simulink model "V2G_Gajduk"  (R2017a)
settings: Solver=ode23t  StartTime=0.0  StopTime=10  RelTol=1e-3
values from neighbouring files (symbols this model uses):
  C_Vdc = 100*18e-3    (= 1.8)    [main_v2gg2v.m]
  Cf = 10*165e-6    (= 0.00165)    [main_v2gg2v.m]
  D = 20    [main_v2gg2v.m]
  E1 = 1.07364213042869    (= 1.07364213043)    [main_v2gg2v.m]
  E2 = 1.05726676017896    (= 1.05726676018)    [main_v2gg2v.m]
  E3 = 1.05298913370226    (= 1.0529891337)    [main_v2gg2v.m]
  f_grid = 50    [main_v2gg2v.m]
  H1 = 10    [main_v2gg2v.m]
  H2 = 15    [main_v2gg2v.m]
  H3 = 60    [main_v2gg2v.m]
  h_PEV = -2000    [main_v2gg2v.m]
  Ibat_ref = -200    [main_v2gg2v.m]
  Ibatfault_ref = 200    [main_v2gg2v.m]
  Ki_CC = 1    [main_v2gg2v.m]
  Ki_inner = 5000    [main_v2gg2v.m]
  Ki_outer = 10000    [main_v2gg2v.m]
  Ki_PLL = 10000    [main_v2gg2v.m]
  Kp_CC = 10    [main_v2gg2v.m]
  Kp_inner = 100    [main_v2gg2v.m]
  Kp_outer = 250    [main_v2gg2v.m]
  Kp_PLL = 100    [main_v2gg2v.m]
  Lbat = 2e-3    (= 0.002)    [main_v2gg2v.m]
  Lgrid = 1/10*0.69e-3    (= 6.9e-05)    [main_v2gg2v.m]
  Linv = 1/10*0.48e-3    (= 4.8e-05)    [main_v2gg2v.m]
  LowSat_CC = 0    [main_v2gg2v.m]
  omega = 2*pi*f_grid    (= 314.159265359)    [main_v2gg2v.m]
  Pm1 = 2.49    [main_v2gg2v.m]
  Pm2 = 4.21    [main_v2gg2v.m]
  Pm3 = 8.20    (= 8.2)    [main_v2gg2v.m]
  Rd = 1.31    [main_v2gg2v.m]
  S1pu = (1.5 + .45j)    [main_v2gg2v.m]
  S2pu = (1.0 + .3j)    [main_v2gg2v.m]
  S3pu = (12.4 + 2.5j)    [main_v2gg2v.m]
  Sbase = 1e6    (= 1000000)    [main_v2gg2v.m]
  Snom_trafo = 1050e6    (= 1050000000)    [main_v2gg2v.m]
  t_fault_end = t_fault_start + FCT    (= 0.723)    [main_v2gg2v.m]
  t_fault_start = 0.5    [main_v2gg2v.m]
  Ts = 1e-5    (= 1e-05)    [main_v2gg2v.m]
  UpSat_CC = 1    [main_v2gg2v.m]
  Vbase = 345e3    (= 345000)    [main_v2gg2v.m]
  Vdc_ref = 1.5e3    (= 1500)    [main_v2gg2v.m]
  Vfault_thresh = 455    [main_v2gg2v.m]
undefined symbols (not defined in the file or in its folder): D1, Delta, Ion, L12, L13, L23, Lbuckboost, Lithium, R_Vdc, Rbuckboost
libraries: powerlib x175, powerlib_meascontrol x55, simulink x45, electricdrivelib x30, dspstat3 x3
(part 5 of 5)

== system V2G_Gajduk/V2G-G2V-3/5 Charging Stations/Charging Station4 ==
  Ibat_ref : Inport
  Battery : electricdrivelib/Extra Sources/Battery  BatType=Lithium-Ion  ShowTempParam=off  ThermalPreset=no  ShowAgeParam=off  NomV=Batt_Vnom  NomQ=Batt_Ah  SOC=Batt_InitSOC  Batt_Tr=Batt_RespTime  PresetModel=on  MaxQ=35  MinV=300  FullV=465.5949  Dis_rate=15.2174  R=0.11429  Normal_OP=31.6522  expZone="[432.1543      1.719565]"  current=[6.5 13 32.5]  Units=Time  Tci=20  NomT=20  T2=-30  MaxQ2=4.8  FullV2=7.1  Normal_OP2=5.655  expZone2="[6.58           1]"  Rca=0.6  ti=2000  Dp=0  Neq0=0  Tsim=1e6  Ta1=25  Qeol=5.4*0.9  Reol=0.013333*1.2  Char_age=[2.3478, 3]  Dis_age=[2.3478, 10]  N1=1500  N2=10500  N3=1000  N4=1400  Ta2=45  N5=950
  Bus Selector : BusSelector  OutputSignals=SOC (%),Current (A),Voltage (V)
  Logical Operator : Logic  Operator=NOT  AllPortsSameDT=off  OutDataTypeStr=boolean
  Mosfet : powerlib/Power Electronics/Mosfet  Ron=0.1  Lon=0  Rd=0.01  Vfd=0  IC=0  Rs=1e5  Cs=inf  Measurements=off
  Mosfet1 : powerlib/Power Electronics/Mosfet  Ron=0.1  Lon=0  Rd=0.01  Vfd=0  IC=0  Rs=1e5  Cs=inf  Measurements=off
  PID Controller4 : simulink/Continuous/PID Controller  Controller=PI  TimeDomain=Continuous-time  SampleTime=-1  IntegratorMethod=Forward Euler  FilterMethod=Forward Euler  Form=Parallel  UseFilter=on  ControllerParametersSource=internal  P=Kp_CC  I=Ki_CC  D=0  N=100  InitialConditionSource=internal  InitialConditionForIntegrator=0  InitialConditionForFilter=0  ExternalReset=none  ZeroCross=off  LimitOutput=on  UpperSaturationLimit=UpSat_CC  LowerSaturationLimit=LowSat_CC  LinearizeAsGain=on  AntiWindupMode=none  Kb=1  TrackingMode=off  Kt=1  PParamMin=[]  PParamMax=[]  IParamMin=[]  IParamMax=[]  DParamMin=[]  DParamMax=[]  NParamMin=[]  NParamMax=[]  KbParamMin=[]  KbParamMax=[]  KtParamMin=[]  KtParamMax=[]  POutMin=[]  POutMax=[]  IOutMin=[]  IOutMax=[]  DOutMin=[]  DOutMax=[]  NOutMin=[]  NOutMax=[]  KbOutMin=[]  KbOutMax=[]  KtOutMin=[]  KtOutMax=[]  IntegratorOutMin=[]  IntegratorOutMax=[]  FilterOutMin=[]  FilterOutMax=[]  SumOutMin=[]  SumOutMax=[]  SumI1OutMin=[]  SumI1OutMax=[]  SumI2OutMin=[]  SumI2OutMax=[]  SumI3OutMin=[]  SumI3OutMax=[]  SumDOutMin=[]  SumDOutMax=[]  SaturationOutMin=[]  SaturationOutMax=[]  IntegratorContinuousStateAttributes=''  IntegratorStateMustResolveToSignalObject=off  IntegratorRTWStateStorageClass=Auto  FilterContinuousStateAttributes=''  FilterStateMustResolveToSignalObject=off  FilterRTWStateStorageClass=Auto  DifferentiatorICPrevScaledInput=0  DifferentiatorOutMin=[]  DifferentiatorOutMax=[]  InitialConditionSetting=State (most efficient)
  PWM Generator (DC-DC) : powerlib_meascontrol/Pulse & Signal Generators/PWM Generator (DC-DC)  Fsw=f_SW  Ts=0
  Series RLC Branch9 : powerlib/Elements/Series RLC Branch  LConnTagsString=__new0  RConnTagsString=__new0  BranchType=L  Resistance=Rbuckboost  Inductance=Lbat  SetiL0=off  InitialCurrent=0  Capacitance=1e-6  Setx0=off  InitialVoltage=0  Measurements=None
  Sum8 : Sum  Inputs=|+-
  Terminator{,1..3} (4 alike) : Terminator
  VDC+ : PMIOPort  Port=1  Side=Left
  VDC- : PMIOPort  Port=2  Side=Left
  wires:
  Bus Selector/3 -> Terminator3/1  "<Voltage (V)>"
  Bus Selector/2 -> Terminator2/1, [Ibat]  "<Current (A)>"
  [Buck] -> Mosfet/1
  Battery/1 -> Terminator/1, Bus Selector/1
  [Boost] -> Mosfet1/1
  Bus Selector/1 -> Terminator1/1  "<SOC (%)>"
  Logical Operator/1 -> [Boost]
  Ibat_ref/1 -> Sum8/2
  PID Controller4/1 -> PWM Generator (DC-DC)/1
  [Ibat] -> Sum8/1
  Sum8/1 -> PID Controller4/1
  PWM Generator (DC-DC)/1 -> Logical Operator/1, [Buck]
  connections:
  VDC-/RConn1 -- Battery/LConn2 -- Mosfet1/RConn1
  Mosfet/LConn1 -- VDC+/RConn1
  Mosfet1/LConn1 -- Series RLC Branch9/RConn1 -- Mosfet/RConn1
  Battery/LConn1 -- Series RLC Branch9/LConn1

== system V2G_Gajduk/V2G-G2V-3/5 Charging Stations/Charging Station5 ==
  Ibat_ref : Inport
  Battery : electricdrivelib/Extra Sources/Battery  BatType=Lithium-Ion  ShowTempParam=off  ThermalPreset=no  ShowAgeParam=off  NomV=Batt_Vnom  NomQ=Batt_Ah  SOC=Batt_InitSOC  Batt_Tr=Batt_RespTime  PresetModel=on  MaxQ=35  MinV=300  FullV=465.5949  Dis_rate=15.2174  R=0.11429  Normal_OP=31.6522  expZone="[432.1543      1.719565]"  current=[6.5 13 32.5]  Units=Time  Tci=20  NomT=20  T2=-30  MaxQ2=4.8  FullV2=7.1  Normal_OP2=5.655  expZone2="[6.58           1]"  Rca=0.6  ti=2000  Dp=0  Neq0=0  Tsim=1e6  Ta1=25  Qeol=5.4*0.9  Reol=0.013333*1.2  Char_age=[2.3478, 3]  Dis_age=[2.3478, 10]  N1=1500  N2=10500  N3=1000  N4=1400  Ta2=45  N5=950
  Bus Selector : BusSelector  OutputSignals=SOC (%),Current (A),Voltage (V)
  Logical Operator : Logic  Operator=NOT  AllPortsSameDT=off  OutDataTypeStr=boolean
  Mosfet : powerlib/Power Electronics/Mosfet  Ron=0.1  Lon=0  Rd=0.01  Vfd=0  IC=0  Rs=1e5  Cs=inf  Measurements=off
  Mosfet1 : powerlib/Power Electronics/Mosfet  Ron=0.1  Lon=0  Rd=0.01  Vfd=0  IC=0  Rs=1e5  Cs=inf  Measurements=off
  PID Controller4 : simulink/Continuous/PID Controller  Controller=PI  TimeDomain=Continuous-time  SampleTime=-1  IntegratorMethod=Forward Euler  FilterMethod=Forward Euler  Form=Parallel  UseFilter=on  ControllerParametersSource=internal  P=Kp_CC  I=Ki_CC  D=0  N=100  InitialConditionSource=internal  InitialConditionForIntegrator=0  InitialConditionForFilter=0  ExternalReset=none  ZeroCross=off  LimitOutput=on  UpperSaturationLimit=UpSat_CC  LowerSaturationLimit=LowSat_CC  LinearizeAsGain=on  AntiWindupMode=none  Kb=1  TrackingMode=off  Kt=1  PParamMin=[]  PParamMax=[]  IParamMin=[]  IParamMax=[]  DParamMin=[]  DParamMax=[]  NParamMin=[]  NParamMax=[]  KbParamMin=[]  KbParamMax=[]  KtParamMin=[]  KtParamMax=[]  POutMin=[]  POutMax=[]  IOutMin=[]  IOutMax=[]  DOutMin=[]  DOutMax=[]  NOutMin=[]  NOutMax=[]  KbOutMin=[]  KbOutMax=[]  KtOutMin=[]  KtOutMax=[]  IntegratorOutMin=[]  IntegratorOutMax=[]  FilterOutMin=[]  FilterOutMax=[]  SumOutMin=[]  SumOutMax=[]  SumI1OutMin=[]  SumI1OutMax=[]  SumI2OutMin=[]  SumI2OutMax=[]  SumI3OutMin=[]  SumI3OutMax=[]  SumDOutMin=[]  SumDOutMax=[]  SaturationOutMin=[]  SaturationOutMax=[]  IntegratorContinuousStateAttributes=''  IntegratorStateMustResolveToSignalObject=off  IntegratorRTWStateStorageClass=Auto  FilterContinuousStateAttributes=''  FilterStateMustResolveToSignalObject=off  FilterRTWStateStorageClass=Auto  DifferentiatorICPrevScaledInput=0  DifferentiatorOutMin=[]  DifferentiatorOutMax=[]  InitialConditionSetting=State (most efficient)
  PWM Generator (DC-DC) : powerlib_meascontrol/Pulse & Signal Generators/PWM Generator (DC-DC)  Fsw=f_SW  Ts=0
  Series RLC Branch9 : powerlib/Elements/Series RLC Branch  LConnTagsString=__new0  RConnTagsString=__new0  BranchType=L  Resistance=Rbuckboost  Inductance=Lbat  SetiL0=off  InitialCurrent=0  Capacitance=1e-6  Setx0=off  InitialVoltage=0  Measurements=None
  Sum8 : Sum  Inputs=|+-
  Terminator{,1..3} (4 alike) : Terminator
  VDC+ : PMIOPort  Port=1  Side=Left
  VDC- : PMIOPort  Port=2  Side=Left
  wires:
  Bus Selector/3 -> Terminator3/1  "<Voltage (V)>"
  Bus Selector/2 -> Terminator2/1, [Ibat]  "<Current (A)>"
  [Buck] -> Mosfet/1
  Battery/1 -> Terminator/1, Bus Selector/1
  [Boost] -> Mosfet1/1
  Bus Selector/1 -> Terminator1/1  "<SOC (%)>"
  Logical Operator/1 -> [Boost]
  Ibat_ref/1 -> Sum8/2
  PID Controller4/1 -> PWM Generator (DC-DC)/1
  [Ibat] -> Sum8/1
  Sum8/1 -> PID Controller4/1
  PWM Generator (DC-DC)/1 -> Logical Operator/1, [Buck]
  connections:
  VDC-/RConn1 -- Battery/LConn2 -- Mosfet1/RConn1
  Mosfet/LConn1 -- VDC+/RConn1
  Mosfet1/LConn1 -- Series RLC Branch9/RConn1 -- Mosfet/RConn1
  Battery/LConn1 -- Series RLC Branch9/LConn1

== system V2G_Gajduk/V2G-G2V-3/5 Charging Stations/Charging Station6 ==
  Ibat_ref : Inport
  Battery : electricdrivelib/Extra Sources/Battery  BatType=Lithium-Ion  ShowTempParam=off  ThermalPreset=no  ShowAgeParam=off  NomV=Batt_Vnom  NomQ=Batt_Ah  SOC=Batt_InitSOC  Batt_Tr=Batt_RespTime  PresetModel=on  MaxQ=35  MinV=300  FullV=465.5949  Dis_rate=15.2174  R=0.11429  Normal_OP=31.6522  expZone="[432.1543      1.719565]"  current=[6.5 13 32.5]  Units=Time  Tci=20  NomT=20  T2=-30  MaxQ2=4.8  FullV2=7.1  Normal_OP2=5.655  expZone2="[6.58           1]"  Rca=0.6  ti=2000  Dp=0  Neq0=0  Tsim=1e6  Ta1=25  Qeol=5.4*0.9  Reol=0.013333*1.2  Char_age=[2.3478, 3]  Dis_age=[2.3478, 10]  N1=1500  N2=10500  N3=1000  N4=1400  Ta2=45  N5=950
  Bus Selector : BusSelector  OutputSignals=SOC (%),Current (A),Voltage (V)
  Logical Operator : Logic  Operator=NOT  AllPortsSameDT=off  OutDataTypeStr=boolean
  Mosfet : powerlib/Power Electronics/Mosfet  Ron=0.1  Lon=0  Rd=0.01  Vfd=0  IC=0  Rs=1e5  Cs=inf  Measurements=off
  Mosfet1 : powerlib/Power Electronics/Mosfet  Ron=0.1  Lon=0  Rd=0.01  Vfd=0  IC=0  Rs=1e5  Cs=inf  Measurements=off
  PID Controller4 : simulink/Continuous/PID Controller  Controller=PI  TimeDomain=Continuous-time  SampleTime=-1  IntegratorMethod=Forward Euler  FilterMethod=Forward Euler  Form=Parallel  UseFilter=on  ControllerParametersSource=internal  P=Kp_CC  I=Ki_CC  D=0  N=100  InitialConditionSource=internal  InitialConditionForIntegrator=0  InitialConditionForFilter=0  ExternalReset=none  ZeroCross=off  LimitOutput=on  UpperSaturationLimit=UpSat_CC  LowerSaturationLimit=LowSat_CC  LinearizeAsGain=on  AntiWindupMode=none  Kb=1  TrackingMode=off  Kt=1  PParamMin=[]  PParamMax=[]  IParamMin=[]  IParamMax=[]  DParamMin=[]  DParamMax=[]  NParamMin=[]  NParamMax=[]  KbParamMin=[]  KbParamMax=[]  KtParamMin=[]  KtParamMax=[]  POutMin=[]  POutMax=[]  IOutMin=[]  IOutMax=[]  DOutMin=[]  DOutMax=[]  NOutMin=[]  NOutMax=[]  KbOutMin=[]  KbOutMax=[]  KtOutMin=[]  KtOutMax=[]  IntegratorOutMin=[]  IntegratorOutMax=[]  FilterOutMin=[]  FilterOutMax=[]  SumOutMin=[]  SumOutMax=[]  SumI1OutMin=[]  SumI1OutMax=[]  SumI2OutMin=[]  SumI2OutMax=[]  SumI3OutMin=[]  SumI3OutMax=[]  SumDOutMin=[]  SumDOutMax=[]  SaturationOutMin=[]  SaturationOutMax=[]  IntegratorContinuousStateAttributes=''  IntegratorStateMustResolveToSignalObject=off  IntegratorRTWStateStorageClass=Auto  FilterContinuousStateAttributes=''  FilterStateMustResolveToSignalObject=off  FilterRTWStateStorageClass=Auto  DifferentiatorICPrevScaledInput=0  DifferentiatorOutMin=[]  DifferentiatorOutMax=[]  InitialConditionSetting=State (most efficient)
  PWM Generator (DC-DC) : powerlib_meascontrol/Pulse & Signal Generators/PWM Generator (DC-DC)  Fsw=f_SW  Ts=0
  Series RLC Branch9 : powerlib/Elements/Series RLC Branch  LConnTagsString=__new0  RConnTagsString=__new0  BranchType=L  Resistance=Rbuckboost  Inductance=Lbat  SetiL0=off  InitialCurrent=0  Capacitance=1e-6  Setx0=off  InitialVoltage=0  Measurements=None
  Sum8 : Sum  Inputs=|+-
  Terminator{,1..3} (4 alike) : Terminator
  VDC+ : PMIOPort  Port=1  Side=Left
  VDC- : PMIOPort  Port=2  Side=Left
  wires:
  Bus Selector/3 -> Terminator3/1  "<Voltage (V)>"
  Bus Selector/2 -> Terminator2/1, [Ibat]  "<Current (A)>"
  [Buck] -> Mosfet/1
  Battery/1 -> Terminator/1, Bus Selector/1
  [Boost] -> Mosfet1/1
  Bus Selector/1 -> Terminator1/1  "<SOC (%)>"
  Logical Operator/1 -> [Boost]
  Ibat_ref/1 -> Sum8/2
  PID Controller4/1 -> PWM Generator (DC-DC)/1
  [Ibat] -> Sum8/1
  Sum8/1 -> PID Controller4/1
  PWM Generator (DC-DC)/1 -> Logical Operator/1, [Buck]
  connections:
  VDC-/RConn1 -- Battery/LConn2 -- Mosfet1/RConn1
  Mosfet/LConn1 -- VDC+/RConn1
  Mosfet1/LConn1 -- Series RLC Branch9/RConn1 -- Mosfet/RConn1
  Battery/LConn1 -- Series RLC Branch9/LConn1

== system V2G_Gajduk/V2G-G2V-3/5 Charging Stations/Charging Station7 ==
  Ibat_ref : Inport
  Battery : electricdrivelib/Extra Sources/Battery  BatType=Lithium-Ion  ShowTempParam=off  ThermalPreset=no  ShowAgeParam=off  NomV=Batt_Vnom  NomQ=Batt_Ah  SOC=Batt_InitSOC  Batt_Tr=Batt_RespTime  PresetModel=on  MaxQ=35  MinV=300  FullV=465.5949  Dis_rate=15.2174  R=0.11429  Normal_OP=31.6522  expZone="[432.1543      1.719565]"  current=[6.5 13 32.5]  Units=Time  Tci=20  NomT=20  T2=-30  MaxQ2=4.8  FullV2=7.1  Normal_OP2=5.655  expZone2="[6.58           1]"  Rca=0.6  ti=2000  Dp=0  Neq0=0  Tsim=1e6  Ta1=25  Qeol=5.4*0.9  Reol=0.013333*1.2  Char_age=[2.3478, 3]  Dis_age=[2.3478, 10]  N1=1500  N2=10500  N3=1000  N4=1400  Ta2=45  N5=950
  Bus Selector : BusSelector  OutputSignals=SOC (%),Current (A),Voltage (V)
  Logical Operator : Logic  Operator=NOT  AllPortsSameDT=off  OutDataTypeStr=boolean
  Mosfet : powerlib/Power Electronics/Mosfet  Ron=0.1  Lon=0  Rd=0.01  Vfd=0  IC=0  Rs=1e5  Cs=inf  Measurements=off
  Mosfet1 : powerlib/Power Electronics/Mosfet  Ron=0.1  Lon=0  Rd=0.01  Vfd=0  IC=0  Rs=1e5  Cs=inf  Measurements=off
  PID Controller4 : simulink/Continuous/PID Controller  Controller=PI  TimeDomain=Continuous-time  SampleTime=-1  IntegratorMethod=Forward Euler  FilterMethod=Forward Euler  Form=Parallel  UseFilter=on  ControllerParametersSource=internal  P=Kp_CC  I=Ki_CC  D=0  N=100  InitialConditionSource=internal  InitialConditionForIntegrator=0  InitialConditionForFilter=0  ExternalReset=none  ZeroCross=off  LimitOutput=on  UpperSaturationLimit=UpSat_CC  LowerSaturationLimit=LowSat_CC  LinearizeAsGain=on  AntiWindupMode=none  Kb=1  TrackingMode=off  Kt=1  PParamMin=[]  PParamMax=[]  IParamMin=[]  IParamMax=[]  DParamMin=[]  DParamMax=[]  NParamMin=[]  NParamMax=[]  KbParamMin=[]  KbParamMax=[]  KtParamMin=[]  KtParamMax=[]  POutMin=[]  POutMax=[]  IOutMin=[]  IOutMax=[]  DOutMin=[]  DOutMax=[]  NOutMin=[]  NOutMax=[]  KbOutMin=[]  KbOutMax=[]  KtOutMin=[]  KtOutMax=[]  IntegratorOutMin=[]  IntegratorOutMax=[]  FilterOutMin=[]  FilterOutMax=[]  SumOutMin=[]  SumOutMax=[]  SumI1OutMin=[]  SumI1OutMax=[]  SumI2OutMin=[]  SumI2OutMax=[]  SumI3OutMin=[]  SumI3OutMax=[]  SumDOutMin=[]  SumDOutMax=[]  SaturationOutMin=[]  SaturationOutMax=[]  IntegratorContinuousStateAttributes=''  IntegratorStateMustResolveToSignalObject=off  IntegratorRTWStateStorageClass=Auto  FilterContinuousStateAttributes=''  FilterStateMustResolveToSignalObject=off  FilterRTWStateStorageClass=Auto  DifferentiatorICPrevScaledInput=0  DifferentiatorOutMin=[]  DifferentiatorOutMax=[]  InitialConditionSetting=State (most efficient)
  PWM Generator (DC-DC) : powerlib_meascontrol/Pulse & Signal Generators/PWM Generator (DC-DC)  Fsw=f_SW  Ts=0
  Series RLC Branch9 : powerlib/Elements/Series RLC Branch  LConnTagsString=__new0  RConnTagsString=__new0  BranchType=L  Resistance=Rbuckboost  Inductance=Lbat  SetiL0=off  InitialCurrent=0  Capacitance=1e-6  Setx0=off  InitialVoltage=0  Measurements=None
  Sum8 : Sum  Inputs=|+-
  Terminator{,1..3} (4 alike) : Terminator
  VDC+ : PMIOPort  Port=1  Side=Left
  VDC- : PMIOPort  Port=2  Side=Left
  wires:
  Bus Selector/3 -> Terminator3/1  "<Voltage (V)>"
  Bus Selector/2 -> Terminator2/1, [Ibat]  "<Current (A)>"
  [Buck] -> Mosfet/1
  Battery/1 -> Terminator/1, Bus Selector/1
  [Boost] -> Mosfet1/1
  Bus Selector/1 -> Terminator1/1  "<SOC (%)>"
  Logical Operator/1 -> [Boost]
  Ibat_ref/1 -> Sum8/2
  PID Controller4/1 -> PWM Generator (DC-DC)/1
  [Ibat] -> Sum8/1
  Sum8/1 -> PID Controller4/1
  PWM Generator (DC-DC)/1 -> Logical Operator/1, [Buck]
  connections:
  VDC-/RConn1 -- Battery/LConn2 -- Mosfet1/RConn1
  Mosfet/LConn1 -- VDC+/RConn1
  Mosfet1/LConn1 -- Series RLC Branch9/RConn1 -- Mosfet/RConn1
  Battery/LConn1 -- Series RLC Branch9/LConn1

== system V2G_Gajduk/V2G-G2V-3/5 Charging Stations/Charging Station8 ==
  Ibat_ref : Inport
  Battery : electricdrivelib/Extra Sources/Battery  BatType=Lithium-Ion  ShowTempParam=off  ThermalPreset=no  ShowAgeParam=off  NomV=Batt_Vnom  NomQ=Batt_Ah  SOC=Batt_InitSOC  Batt_Tr=Batt_RespTime  PresetModel=on  MaxQ=35  MinV=300  FullV=465.5949  Dis_rate=15.2174  R=0.11429  Normal_OP=31.6522  expZone="[432.1543      1.719565]"  current=[6.5 13 32.5]  Units=Time  Tci=20  NomT=20  T2=-30  MaxQ2=4.8  FullV2=7.1  Normal_OP2=5.655  expZone2="[6.58           1]"  Rca=0.6  ti=2000  Dp=0  Neq0=0  Tsim=1e6  Ta1=25  Qeol=5.4*0.9  Reol=0.013333*1.2  Char_age=[2.3478, 3]  Dis_age=[2.3478, 10]  N1=1500  N2=10500  N3=1000  N4=1400  Ta2=45  N5=950
  Bus Selector : BusSelector  OutputSignals=SOC (%),Current (A),Voltage (V)
  Logical Operator : Logic  Operator=NOT  AllPortsSameDT=off  OutDataTypeStr=boolean
  Mosfet : powerlib/Power Electronics/Mosfet  Ron=0.1  Lon=0  Rd=0.01  Vfd=0  IC=0  Rs=1e5  Cs=inf  Measurements=off
  Mosfet1 : powerlib/Power Electronics/Mosfet  Ron=0.1  Lon=0  Rd=0.01  Vfd=0  IC=0  Rs=1e5  Cs=inf  Measurements=off
  PID Controller4 : simulink/Continuous/PID Controller  Controller=PI  TimeDomain=Continuous-time  SampleTime=-1  IntegratorMethod=Forward Euler  FilterMethod=Forward Euler  Form=Parallel  UseFilter=on  ControllerParametersSource=internal  P=Kp_CC  I=Ki_CC  D=0  N=100  InitialConditionSource=internal  InitialConditionForIntegrator=0  InitialConditionForFilter=0  ExternalReset=none  ZeroCross=off  LimitOutput=on  UpperSaturationLimit=UpSat_CC  LowerSaturationLimit=LowSat_CC  LinearizeAsGain=on  AntiWindupMode=none  Kb=1  TrackingMode=off  Kt=1  PParamMin=[]  PParamMax=[]  IParamMin=[]  IParamMax=[]  DParamMin=[]  DParamMax=[]  NParamMin=[]  NParamMax=[]  KbParamMin=[]  KbParamMax=[]  KtParamMin=[]  KtParamMax=[]  POutMin=[]  POutMax=[]  IOutMin=[]  IOutMax=[]  DOutMin=[]  DOutMax=[]  NOutMin=[]  NOutMax=[]  KbOutMin=[]  KbOutMax=[]  KtOutMin=[]  KtOutMax=[]  IntegratorOutMin=[]  IntegratorOutMax=[]  FilterOutMin=[]  FilterOutMax=[]  SumOutMin=[]  SumOutMax=[]  SumI1OutMin=[]  SumI1OutMax=[]  SumI2OutMin=[]  SumI2OutMax=[]  SumI3OutMin=[]  SumI3OutMax=[]  SumDOutMin=[]  SumDOutMax=[]  SaturationOutMin=[]  SaturationOutMax=[]  IntegratorContinuousStateAttributes=''  IntegratorStateMustResolveToSignalObject=off  IntegratorRTWStateStorageClass=Auto  FilterContinuousStateAttributes=''  FilterStateMustResolveToSignalObject=off  FilterRTWStateStorageClass=Auto  DifferentiatorICPrevScaledInput=0  DifferentiatorOutMin=[]  DifferentiatorOutMax=[]  InitialConditionSetting=State (most efficient)
  PWM Generator (DC-DC) : powerlib_meascontrol/Pulse & Signal Generators/PWM Generator (DC-DC)  Fsw=f_SW  Ts=0
  Series RLC Branch9 : powerlib/Elements/Series RLC Branch  LConnTagsString=__new0  RConnTagsString=__new0  BranchType=L  Resistance=Rbuckboost  Inductance=Lbat  SetiL0=off  InitialCurrent=0  Capacitance=1e-6  Setx0=off  InitialVoltage=0  Measurements=None
  Sum8 : Sum  Inputs=|+-
  Terminator{,1..3} (4 alike) : Terminator
  VDC+ : PMIOPort  Port=1  Side=Left
  VDC- : PMIOPort  Port=2  Side=Left
  wires:
  Bus Selector/3 -> Terminator3/1  "<Voltage (V)>"
  Bus Selector/2 -> Terminator2/1, [Ibat]  "<Current (A)>"
  [Buck] -> Mosfet/1
  Battery/1 -> Terminator/1, Bus Selector/1
  [Boost] -> Mosfet1/1
  Bus Selector/1 -> Terminator1/1  "<SOC (%)>"
  Logical Operator/1 -> [Boost]
  Ibat_ref/1 -> Sum8/2
  PID Controller4/1 -> PWM Generator (DC-DC)/1
  [Ibat] -> Sum8/1
  Sum8/1 -> PID Controller4/1
  PWM Generator (DC-DC)/1 -> Logical Operator/1, [Buck]
  connections:
  VDC-/RConn1 -- Battery/LConn2 -- Mosfet1/RConn1
  Mosfet/LConn1 -- VDC+/RConn1
  Mosfet1/LConn1 -- Series RLC Branch9/RConn1 -- Mosfet/RConn1
  Battery/LConn1 -- Series RLC Branch9/LConn1

== system V2G_Gajduk/V2G-G2V-3/5 Charging Stations/Charging Station9 ==
  Ibat_ref : Inport
  Battery : electricdrivelib/Extra Sources/Battery  BatType=Lithium-Ion  ShowTempParam=off  ThermalPreset=no  ShowAgeParam=off  NomV=Batt_Vnom  NomQ=Batt_Ah  SOC=Batt_InitSOC  Batt_Tr=Batt_RespTime  PresetModel=on  MaxQ=35  MinV=300  FullV=465.5949  Dis_rate=15.2174  R=0.11429  Normal_OP=31.6522  expZone="[432.1543      1.719565]"  current=[6.5 13 32.5]  Units=Time  Tci=20  NomT=20  T2=-30  MaxQ2=4.8  FullV2=7.1  Normal_OP2=5.655  expZone2="[6.58           1]"  Rca=0.6  ti=2000  Dp=0  Neq0=0  Tsim=1e6  Ta1=25  Qeol=5.4*0.9  Reol=0.013333*1.2  Char_age=[2.3478, 3]  Dis_age=[2.3478, 10]  N1=1500  N2=10500  N3=1000  N4=1400  Ta2=45  N5=950
  Bus Selector : BusSelector  OutputSignals=SOC (%),Current (A),Voltage (V)
  Logical Operator : Logic  Operator=NOT  AllPortsSameDT=off  OutDataTypeStr=boolean
  Mosfet : powerlib/Power Electronics/Mosfet  Ron=0.1  Lon=0  Rd=0.01  Vfd=0  IC=0  Rs=1e5  Cs=inf  Measurements=off
  Mosfet1 : powerlib/Power Electronics/Mosfet  Ron=0.1  Lon=0  Rd=0.01  Vfd=0  IC=0  Rs=1e5  Cs=inf  Measurements=off
  PID Controller4 : simulink/Continuous/PID Controller  Controller=PI  TimeDomain=Continuous-time  SampleTime=-1  IntegratorMethod=Forward Euler  FilterMethod=Forward Euler  Form=Parallel  UseFilter=on  ControllerParametersSource=internal  P=Kp_CC  I=Ki_CC  D=0  N=100  InitialConditionSource=internal  InitialConditionForIntegrator=0  InitialConditionForFilter=0  ExternalReset=none  ZeroCross=off  LimitOutput=on  UpperSaturationLimit=UpSat_CC  LowerSaturationLimit=LowSat_CC  LinearizeAsGain=on  AntiWindupMode=none  Kb=1  TrackingMode=off  Kt=1  PParamMin=[]  PParamMax=[]  IParamMin=[]  IParamMax=[]  DParamMin=[]  DParamMax=[]  NParamMin=[]  NParamMax=[]  KbParamMin=[]  KbParamMax=[]  KtParamMin=[]  KtParamMax=[]  POutMin=[]  POutMax=[]  IOutMin=[]  IOutMax=[]  DOutMin=[]  DOutMax=[]  NOutMin=[]  NOutMax=[]  KbOutMin=[]  KbOutMax=[]  KtOutMin=[]  KtOutMax=[]  IntegratorOutMin=[]  IntegratorOutMax=[]  FilterOutMin=[]  FilterOutMax=[]  SumOutMin=[]  SumOutMax=[]  SumI1OutMin=[]  SumI1OutMax=[]  SumI2OutMin=[]  SumI2OutMax=[]  SumI3OutMin=[]  SumI3OutMax=[]  SumDOutMin=[]  SumDOutMax=[]  SaturationOutMin=[]  SaturationOutMax=[]  IntegratorContinuousStateAttributes=''  IntegratorStateMustResolveToSignalObject=off  IntegratorRTWStateStorageClass=Auto  FilterContinuousStateAttributes=''  FilterStateMustResolveToSignalObject=off  FilterRTWStateStorageClass=Auto  DifferentiatorICPrevScaledInput=0  DifferentiatorOutMin=[]  DifferentiatorOutMax=[]  InitialConditionSetting=State (most efficient)
  PWM Generator (DC-DC) : powerlib_meascontrol/Pulse & Signal Generators/PWM Generator (DC-DC)  Fsw=f_SW  Ts=0
  Series RLC Branch9 : powerlib/Elements/Series RLC Branch  LConnTagsString=__new0  RConnTagsString=__new0  BranchType=L  Resistance=Rbuckboost  Inductance=Lbat  SetiL0=off  InitialCurrent=0  Capacitance=1e-6  Setx0=off  InitialVoltage=0  Measurements=None
  Sum8 : Sum  Inputs=|+-
  Terminator{,1..3} (4 alike) : Terminator
  VDC+ : PMIOPort  Port=1  Side=Left
  VDC- : PMIOPort  Port=2  Side=Left
  wires:
  Bus Selector/3 -> Terminator3/1  "<Voltage (V)>"
  Bus Selector/2 -> Terminator2/1, [Ibat]  "<Current (A)>"
  [Buck] -> Mosfet/1
  Battery/1 -> Terminator/1, Bus Selector/1
  [Boost] -> Mosfet1/1
  Bus Selector/1 -> Terminator1/1  "<SOC (%)>"
  Logical Operator/1 -> [Boost]
  Ibat_ref/1 -> Sum8/2
  PID Controller4/1 -> PWM Generator (DC-DC)/1
  [Ibat] -> Sum8/1
  Sum8/1 -> PID Controller4/1
  PWM Generator (DC-DC)/1 -> Logical Operator/1, [Buck]
  connections:
  VDC-/RConn1 -- Battery/LConn2 -- Mosfet1/RConn1
  Mosfet/LConn1 -- VDC+/RConn1
  Mosfet1/LConn1 -- Series RLC Branch9/RConn1 -- Mosfet/RConn1
  Battery/LConn1 -- Series RLC Branch9/LConn1

== system V2G_Gajduk/V2G-G2V-3/AC//DC Converter/Subsystem ==
  PWM1 : Inport
  PWM2 : Inport  Port=2
  PWM3 : Inport  Port=3
  PWM4 : Inport  Port=4
  PWM5 : Inport  Port=5
  PWM6 : Inport  Port=6
  IGBT/Diode{,1..5} (6 alike) : powerlib/Power Electronics/IGBT//Diode  Ron=1e-3  Rs=1e5  Cs=inf  Measurements=off
  VR : PMIOPort  Port=1  Side=Left
  VY : PMIOPort  Port=2  Side=Left
  VB : PMIOPort  Port=3  Side=Left
  VDC+ : PMIOPort  Port=4  Side=Right
  VDC- : PMIOPort  Port=5  Side=Right
  wires:
  PWM1/1 -> IGBT/Diode/1
  PWM5/1 -> IGBT/Diode4/1
  PWM4/1 -> IGBT/Diode3/1
  PWM6/1 -> IGBT/Diode5/1
  PWM3/1 -> IGBT/Diode2/1
  PWM2/1 -> IGBT/Diode1/1
  connections:
  IGBT/Diode4/RConn1 -- VB/RConn1 -- IGBT/Diode5/LConn1
  IGBT/Diode1/RConn1 -- IGBT/Diode3/RConn1 -- VDC-/RConn1 -- IGBT/Diode5/RConn1
  IGBT/Diode/RConn1 -- VR/RConn1 -- IGBT/Diode1/LConn1
  IGBT/Diode2/RConn1 -- VY/RConn1 -- IGBT/Diode3/LConn1
  IGBT/Diode/LConn1 -- VDC+/RConn1 -- IGBT/Diode4/LConn1 -- IGBT/Diode2/LConn1

== matlab function V2G_Gajduk/V2G-G2V-1/MovingRMSFaultDetect1/MATLAB Function ==
  data: first_fault input; v input; t input; y output; first_fault output; Ibat_ref input; Vfault_thresh input
function [y, first_fault] = fcn(first_fault,v,t, Ibat_ref, Vfault_thresh)
if (v < Vfault_thresh && t > 0.2)
    first_fault = true;
end
if(first_fault)
    y = Ibat_ref;
else
    y = 0;
end

end

== matlab function V2G_Gajduk/V2G-G2V-2/MovingRMSFaultDetect2/MATLAB Function ==
  data: first_fault input; v input; t input; y output; first_fault output; Ibat_ref input; Vfault_thresh input
function [y, first_fault] = fcn(first_fault,v,t, Ibat_ref, Vfault_thresh)
if (v < Vfault_thresh && t > 0.2)
    first_fault = true;
end
if(first_fault)
    y = Ibat_ref;
else
    y = 0;
end

end

== matlab function V2G_Gajduk/V2G-G2V-3/MovingRMSFaultDetect2/MATLAB Function ==
  data: first_fault input; v input; t input; y output; first_fault output; Ibat_ref input; Vfault_thresh input
function [y, first_fault] = fcn(first_fault,v,t, Ibat_ref, Vfault_thresh)
if (v < Vfault_thresh && t > 0.2)
    first_fault = true;
end
if(first_fault)
    y = Ibat_ref;
else
    y = 0;
end

end
